simulink model "un_tanque"  (R2016a)
settings: Solver=ode23tb  StartTime=0.0  StopTime=30.0  RelTol=1e-3
settings Model: Creator=Matias  LastModifiedBy=Matias

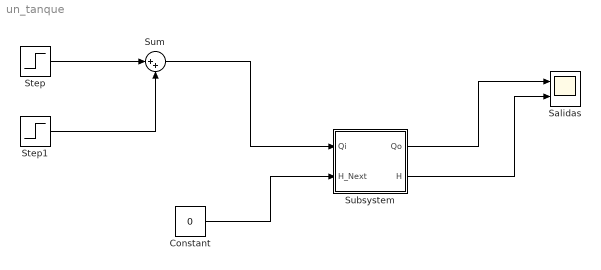
== system un_tanque ==
  Constant : Constant  Value=0
  Salidas : Scope  NumInputPorts=2
  Step : Step  SampleTime=0
  Step1 : Step  Time=15  After=-1  SampleTime=0
  Subsystem : Subsystem
  Sum : Sum  Inputs=|++
  wires:
  Constant/1 -> Subsystem/2(H_Next)
  Subsystem/1(Qo) -> Salidas/1
  Step/1 -> Sum/1
  Sum/1 -> Subsystem/1("Qi ")
  Step1/1 -> Sum/2
  Subsystem/2("H ") -> Salidas/2

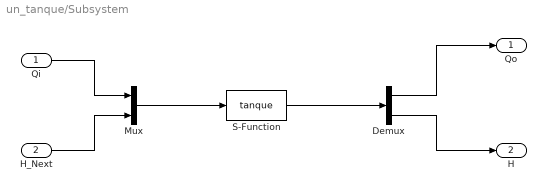
== system un_tanque/Subsystem ==
  "Qi " : Inport
  H_Next : Inport  Port=2
  Demux : Demux  Outputs=2
  Mux : Mux  Inputs=2
  S-Function : S-Function  FunctionName=tanque  Parameters=1, 0.75, 1, 0  SFunctionDeploymentMode=off  EnableBusSupport=off
  Qo : Outport
  "H " : Outport  Port=2
  wires:
  Mux/1 -> S-Function/1
  "Qi "/1 -> Mux/1
  H_Next/1 -> Mux/2
  S-Function/1 -> Demux/1
  Demux/2 -> "H "/1
  Demux/1 -> Qo/1
